simulink subsystem "IMU"  (R2024b)
settings: Solver=VariableStepAuto  StartTime=0.0  StopTime=10.0  RelTol=1e-3
settings Model: Creator=JesseJabezArendse  LastModifiedBy=JesseJabezArendse
settings RTWCC: GPUComputeCapability=3.5

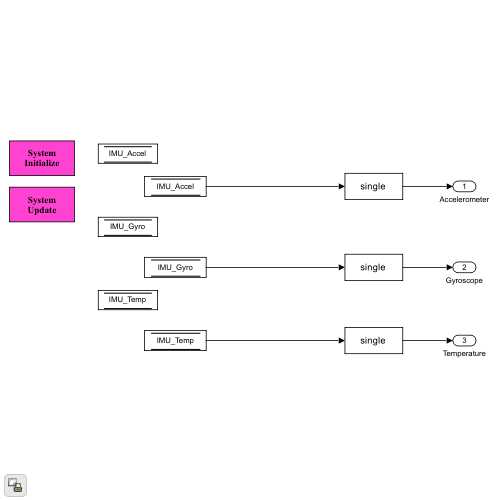
[thumbnail: Simulink's stored preview of the top-level diagram]
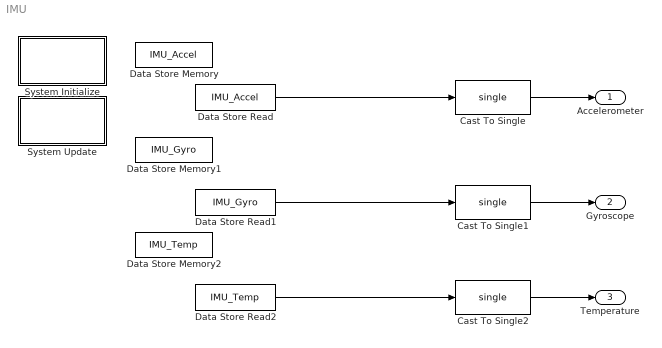
== system IMU ==
  Cast To Single : DataTypeConversion  OutDataTypeStr=single  SaturateOnIntegerOverflow=off  RndMeth=Floor
  Cast To Single1 : DataTypeConversion  OutDataTypeStr=single  SaturateOnIntegerOverflow=off  RndMeth=Floor
  Cast To Single2 : DataTypeConversion  OutDataTypeStr=single  SaturateOnIntegerOverflow=off  RndMeth=Floor
  Data Store Memory : DataStoreMemory  DataStoreName=IMU_Accel  WriteAfterWriteMsg=warning  ShowAdditionalParam=off  OutDataTypeStr=single  Dimensions=3
  Data Store Memory1 : DataStoreMemory  DataStoreName=IMU_Gyro  WriteAfterWriteMsg=warning  ShowAdditionalParam=off  OutDataTypeStr=single  Dimensions=3
  Data Store Memory2 : DataStoreMemory  DataStoreName=IMU_Temp  WriteAfterWriteMsg=warning  ShowAdditionalParam=off  OutDataTypeStr=single  Dimensions=1
  Data Store Read : DataStoreRead  DataStoreName=IMU_Accel  IndexOptions=Index vector (dialog)  Indices=1  OutputSizes=1
  Data Store Read1 : DataStoreRead  DataStoreName=IMU_Gyro  IndexOptions=Index vector (dialog)  Indices=1  OutputSizes=1
  Data Store Read2 : DataStoreRead  DataStoreName=IMU_Temp  IndexOptions=Index vector (dialog)  Indices=1  OutputSizes=1
  System Initialize : Subsystem  mask(System Initialize){ShowInLibBrowser=0}
      mask prompts: ShowInLibBrowser "Simulink:masks:CustCodeMaskParam1_MP"
      settings: CopyFcn=cccopyfcn(gcb)  OpenFcn=ccopenfcn('System Initialize Function')
      mask Help: eval('feval(''rtwprivate'',''rtwhelpview'',''rtw_sys_initialize_block'')');
      mask Display: disp('System\nInitialize');
  System Update : Subsystem  mask(System Update){ShowInLibBrowser=0}
      mask prompts: ShowInLibBrowser "Simulink:masks:CustCodeMaskParam1_MP"
      settings: CopyFcn=cccopyfcn(gcb)  OpenFcn=ccopenfcn('System Update Function')
      mask Help: eval('feval(''rtwprivate'',''rtwhelpview'',''rtw_sys_update_block'')');
      mask Display: disp('System\nUpdate');
  Accelerometer : Outport  OutDataTypeStr=single  PortDimensions=3
  Gyroscope : Outport  Port=2  OutDataTypeStr=single  PortDimensions=3
  Temperature : Outport  Port=3  OutDataTypeStr=single  PortDimensions=1
  wires:
  Data Store Read/1 -> Cast To Single/1
  Data Store Read1/1 -> Cast To Single1/1
  Cast To Single/1 -> Accelerometer/1
  Cast To Single1/1 -> Gyroscope/1
  Data Store Read2/1 -> Cast To Single2/1
  Cast To Single2/1 -> Temperature/1

== system IMU/System Initialize ==

== system IMU/System Update ==
